simulink model "RadarSimulinkProjectRev009"  (R2024a)
settings: Solver=VariableStepAuto  StartTime=0.0  StopTime=0.0125  RelTol=1e-3
values from neighbouring files (symbols this model uses):
  AngleTime = SweepTime/10    (= 10000)    [InitializationOfVariables.m]    (also in InitializationOfVariablesRev000.m; InitializationOfVariablesRev001.m; InitializationOfVariablesRev003.m = 2097152; InitializationOfVariablesRev004.m = 2097152)
  ASR_LUT = Rsamp-OffsetDelayR    [InitializationOfVariablesRev003.m]    (also in InitializationOfVariablesRev004.m = round((R*2*SystemFs)/c))
  Btn_Debounce = 20000    [InitializationOfVariablesRev003.m]    (also in InitializationOfVariablesRev004.m)
  ChirpNc = 128    [InitializationOfVariablesRev003.m]    (also in InitializationOfVariablesRev004.m)
  ChirpSizeLength = FreqDeltaPeriod*361    (= 16245)    [InitializationOfVariablesRev003.m]    (also in InitializationOfVariablesRev004.m = 16384)
  DeciFactor = 8    [InitializationOfVariablesRev004.m]
  FCW = [FCW_p1, FCW_p2]    [InitializationOfVariablesRev003.m]    (also in InitializationOfVariablesRev004.m = f / SystemFs)
  RXFFTLength = 16384    [InitializationOfVariablesRev003.m]    (also in InitializationOfVariablesRev004.m = 2048)
  SweepTime = 100000    [InitializationOfVariables.m]    (also in InitializationOfVariablesRev000.m; InitializationOfVariablesRev001.m; InitializationOfVariablesRev003.m = 23068672; InitializationOfVariablesRev004.m = 23068672)
undefined symbols (not defined in the file or in its folder): SignalGenerationForAnalysis, Subsystem, xc7a200tfbg676
libraries: hdlBasic x407, hdlUtilities x11, hdlDSPIP x11, vmcUtilities x1
(part 4 of 4)

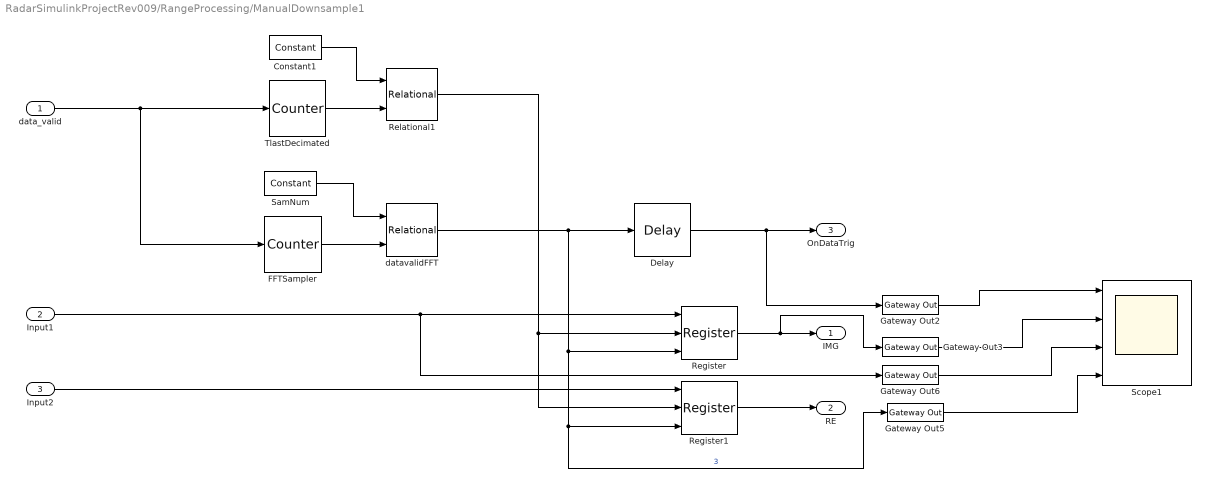
== system RadarSimulinkProjectRev009/RangeProcessing/ManualDownsample1 ==
  data_valid : Inport
  Input1 : Inport  Port=2
  Input2 : Inport  Port=3
  Constant1 : hdlBasic/Constant  const=RXFFTLength*8-1  gui_display_data_type=Fixed-point  arith_type=Signed (2's comp)  n_bits=16  bin_pt=0  preci_type=Single  exp_width=8  frac_width=24  explicit_period=off  period=1  XmcBlockStatus=1  maskContainerNames=tabcontainer1  block_type=constant  block_config=sysgen:Constant_config
  Delay : hdlBasic/Delay  rst=off  en=off  latency=1  reg_retiming=off  XmcBlockStatus=1  maskContainerNames=group1  block_type=delay  block_config=sysgen:Delay_config
  FFTSampler : hdlBasic/Counter  cnt_type=Count limited  cnt_to=DeciFactor-1  operation=Up  start_count=0  cnt_by_val=1  arith_type=Unsigned  n_bits=4  bin_pt=0  load_pin=off  rst=off  en=on  explicit_period=Explicit  period=P1  use_behavioral_HDL=off  implementation=Fabric  XmcBlockStatus=1  maskContainerNames=group1  block_type=counter  block_config=sysgen:Counter_config  block_width=531  block_height=1023
  Gateway Out{2..3,5..6} (4 alike) : hdlBasic/Gateway Out  inherit_from_input=off  bool_to_boolean=off  hdl_port=on  rows=1  columns=1  UseAsDAC=off  DACChannel='1'  interface=None  automatic_assignment=on  address_offset=hex2dec('00')  intf_name=''  intf_description=''  timing_constraint=None  locs_specified=off  LOCs={}  io_standard={}  XmcBlockStatus=1  maskContainerNames=group4  block_type=gatewayout  block_config=sysgen:gateway_out_config  block_width_w=590  block_height_w=620  block_width=620  block_height=750
  Register : hdlBasic/Register  init=0  rst=on  en=on  XmcBlockStatus=1  maskContainerNames=tabcontainer1  block_type=register  block_config=sysgen:Register_config
  Register1 : hdlBasic/Register  init=0  rst=on  en=on  XmcBlockStatus=1  maskContainerNames=tabcontainer1  block_type=register  block_config=sysgen:Register_config
  Relational1 : hdlBasic/Relational  mode=a=b  op_type=Bool  en=off  latency=0  XmcBlockStatus=1  maskContainerNames=tabcontainer1  block_type=relational  block_config=sysgen:Relational_config
  SamNum : hdlBasic/Constant  const=5  gui_display_data_type=Fixed-point  arith_type=Signed (2's comp)  n_bits=5  bin_pt=0  preci_type=Single  exp_width=8  frac_width=24  explicit_period=off  period=1  XmcBlockStatus=1  maskContainerNames=tabcontainer1  block_type=constant  block_config=sysgen:Constant_config
  Scope1 : Scope  NumInputPorts=4
  TlastDecimated : hdlBasic/Counter  cnt_type=Count limited  cnt_to=2047  operation=Up  start_count=0  cnt_by_val=1  arith_type=Unsigned  n_bits=12  bin_pt=0  load_pin=off  rst=off  en=on  explicit_period=Inferred from inputs  period=P1  use_behavioral_HDL=off  implementation=Fabric  XmcBlockStatus=1  maskContainerNames=group1  block_type=counter  block_config=sysgen:Counter_config  block_width=531  block_height=1023
  datavalidFFT : hdlBasic/Relational  mode=a=b  op_type=Bool  en=off  latency=0  XmcBlockStatus=1  maskContainerNames=tabcontainer1  block_type=relational  block_config=sysgen:Relational_config
  IMG : Outport
  RE : Outport  Port=2
  OnDataTrig : Outport  Port=3
  wires:
  data_valid/1 -> FFTSampler/1, TlastDecimated/1
  Constant1/1 -> Relational1/1
  FFTSampler/1 -> datavalidFFT/2
  datavalidFFT/1 -> Gateway Out5/1, Register1/3, Register/3, Delay/1  "3"
  TlastDecimated/1 -> Relational1/2
  SamNum/1 -> datavalidFFT/1
  Register/1 -> Gateway Out3/1, IMG/1
  Register1/1 -> RE/1
  Delay/1 -> Gateway Out2/1, OnDataTrig/1
  Input1/1 -> Gateway Out6/1, Register/1
  Input2/1 -> Register1/1
  Relational1/1 -> Register/2, Register1/2
  Gateway Out3/1 -> Scope1/2
  Gateway Out6/1 -> Scope1/3
  Gateway Out5/1 -> Scope1/4
  Gateway Out2/1 -> Scope1/1

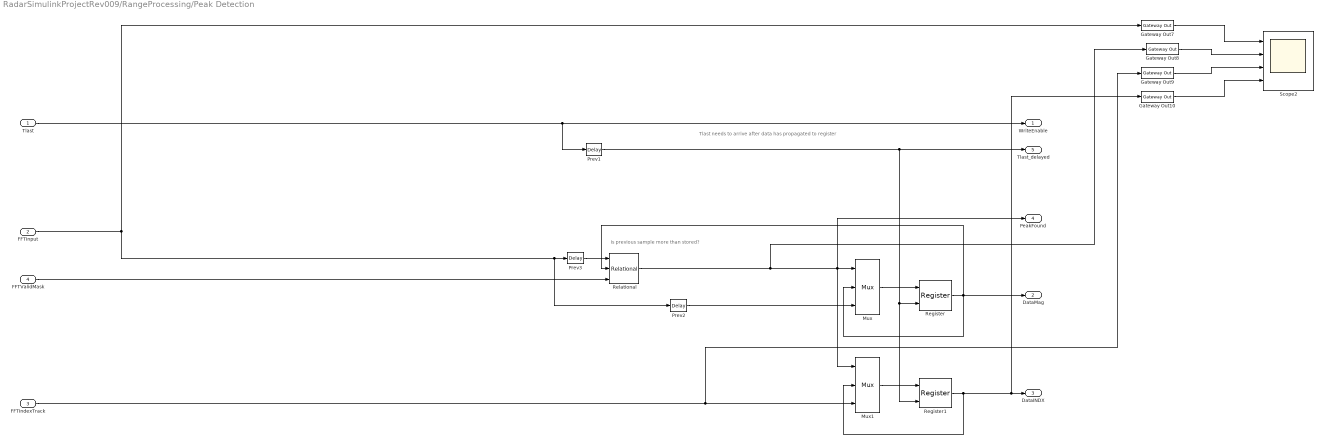
== system RadarSimulinkProjectRev009/RangeProcessing/Peak Detection ==
  note: Tlast needs to arrive after data has propagated to register
  note: Is previous sample more than stored?
  Tlast : Inport
  FFTInput : Inport  Port=2
  FFTIndexTrack : Inport  Port=3
  FFTValidMask : Inport  Port=4
  Gateway Out{7..10} (4 alike) : hdlBasic/Gateway Out  inherit_from_input=off  bool_to_boolean=off  hdl_port=on  rows=1  columns=1  UseAsDAC=off  DACChannel='1'  interface=None  automatic_assignment=on  address_offset=hex2dec('00')  intf_name=''  intf_description=''  timing_constraint=None  locs_specified=off  LOCs={}  io_standard={}  XmcBlockStatus=1  maskContainerNames=group4  block_type=gatewayout  block_config=sysgen:gateway_out_config  block_width_w=590  block_height_w=620  block_width=620  block_height=750
  Mux : hdlBasic/Mux  inputs=2  en=off  latency=0  precision=Full  arith_type=Unsigned  n_bits=16  bin_pt=14  quantization=Truncate  overflow=Wrap  XmcBlockStatus=1  maskContainerNames=tabcontainer1  block_type=mux  block_config=sysgen:Mux_config
  Mux1 : hdlBasic/Mux  inputs=2  en=off  latency=0  precision=Full  arith_type=Unsigned  n_bits=16  bin_pt=14  quantization=Truncate  overflow=Wrap  XmcBlockStatus=1  maskContainerNames=tabcontainer1  block_type=mux  block_config=sysgen:Mux_config
  Prev1 : hdlBasic/Delay  rst=off  en=off  latency=4  reg_retiming=off  XmcBlockStatus=1  maskContainerNames=group1  block_type=delay  block_config=sysgen:Delay_config
  Prev2 : hdlBasic/Delay  rst=off  en=off  latency=2  reg_retiming=off  XmcBlockStatus=1  maskContainerNames=group1  block_type=delay  block_config=sysgen:Delay_config
  Prev3 : hdlBasic/Delay  rst=off  en=off  latency=1  reg_retiming=off  XmcBlockStatus=1  maskContainerNames=group1  block_type=delay  block_config=sysgen:Delay_config
  Register : hdlBasic/Register  init=0  rst=on  en=off  XmcBlockStatus=1  maskContainerNames=tabcontainer1  block_type=register  block_config=sysgen:Register_config
  Register1 : hdlBasic/Register  init=0  rst=on  en=off  XmcBlockStatus=1  maskContainerNames=tabcontainer1  block_type=register  block_config=sysgen:Register_config
  Relational : hdlBasic/Relational  mode=a>b  op_type=Bool  en=on  latency=1  XmcBlockStatus=1  maskContainerNames=tabcontainer1  block_type=relational  block_config=sysgen:Relational_config
  Scope2 : Scope  NumInputPorts=4
  WriteEnable : Outport
  DataMag : Outport  Port=2
  DataINDX : Outport  Port=3
  PeakFound : Outport  Port=4
  Tlast_delayed : Outport  Port=5
  wires:
  FFTValidMask/1 -> Relational/3
  Tlast/1 -> Prev1/1, WriteEnable/1
  Prev2/1 -> Mux/3
  Register/1 -> Relational/2, DataMag/1, Mux/2
  Mux/1 -> Register/1
  Register1/1 -> Gateway Out10/1, DataINDX/1, Mux1/2
  FFTIndexTrack/1 -> Gateway Out9/1, Mux1/3
  Mux1/1 -> Register1/1
  Prev1/1 -> Register1/2, Register/2, Tlast_delayed/1
  Gateway Out7/1 -> Scope2/1
  Gateway Out8/1 -> Scope2/2
  Gateway Out9/1 -> Scope2/3
  Gateway Out10/1 -> Scope2/4
  FFTInput/1 -> Gateway Out7/1, Prev3/1, Prev2/1
  Prev3/1 -> Relational/1
  Relational/1 -> Gateway Out8/1, Mux1/1, Mux/1, PeakFound/1

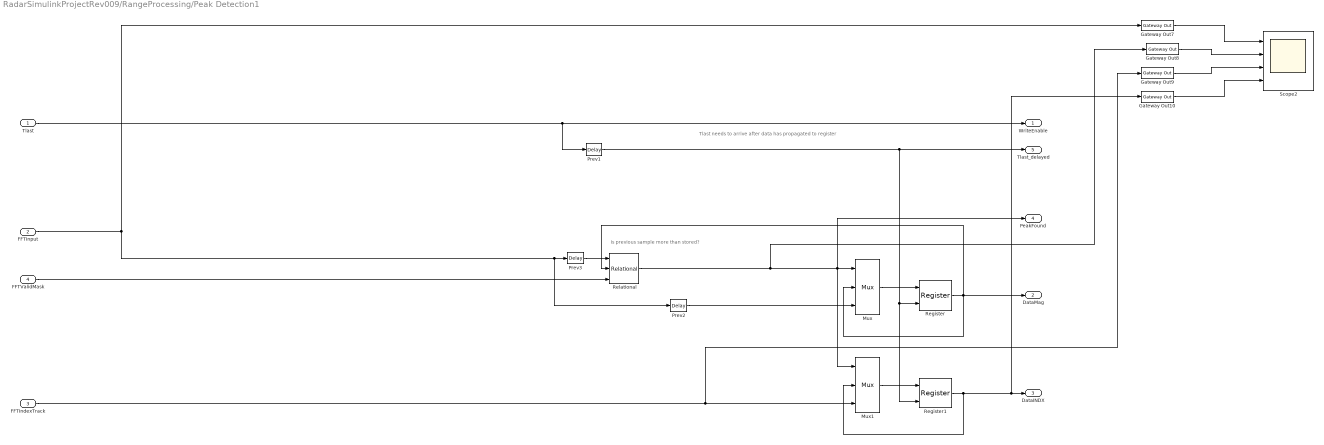
== system RadarSimulinkProjectRev009/RangeProcessing/Peak Detection1 ==
  note: Tlast needs to arrive after data has propagated to register
  note: Is previous sample more than stored?
  Tlast : Inport
  FFTInput : Inport  Port=2
  FFTIndexTrack : Inport  Port=3
  FFTValidMask : Inport  Port=4
  Gateway Out{7..10} (4 alike) : hdlBasic/Gateway Out  inherit_from_input=off  bool_to_boolean=off  hdl_port=on  rows=1  columns=1  UseAsDAC=off  DACChannel='1'  interface=None  automatic_assignment=on  address_offset=hex2dec('00')  intf_name=''  intf_description=''  timing_constraint=None  locs_specified=off  LOCs={}  io_standard={}  XmcBlockStatus=1  maskContainerNames=group4  block_type=gatewayout  block_config=sysgen:gateway_out_config  block_width_w=590  block_height_w=620  block_width=620  block_height=750
  Mux : hdlBasic/Mux  inputs=2  en=off  latency=0  precision=Full  arith_type=Unsigned  n_bits=16  bin_pt=14  quantization=Truncate  overflow=Wrap  XmcBlockStatus=1  maskContainerNames=tabcontainer1  block_type=mux  block_config=sysgen:Mux_config
  Mux1 : hdlBasic/Mux  inputs=2  en=off  latency=0  precision=Full  arith_type=Unsigned  n_bits=16  bin_pt=14  quantization=Truncate  overflow=Wrap  XmcBlockStatus=1  maskContainerNames=tabcontainer1  block_type=mux  block_config=sysgen:Mux_config
  Prev1 : hdlBasic/Delay  rst=off  en=off  latency=4  reg_retiming=off  XmcBlockStatus=1  maskContainerNames=group1  block_type=delay  block_config=sysgen:Delay_config
  Prev2 : hdlBasic/Delay  rst=off  en=off  latency=2  reg_retiming=off  XmcBlockStatus=1  maskContainerNames=group1  block_type=delay  block_config=sysgen:Delay_config
  Prev3 : hdlBasic/Delay  rst=off  en=off  latency=1  reg_retiming=off  XmcBlockStatus=1  maskContainerNames=group1  block_type=delay  block_config=sysgen:Delay_config
  Register : hdlBasic/Register  init=0  rst=on  en=off  XmcBlockStatus=1  maskContainerNames=tabcontainer1  block_type=register  block_config=sysgen:Register_config
  Register1 : hdlBasic/Register  init=0  rst=on  en=off  XmcBlockStatus=1  maskContainerNames=tabcontainer1  block_type=register  block_config=sysgen:Register_config
  Relational : hdlBasic/Relational  mode=a>b  op_type=Bool  en=on  latency=1  XmcBlockStatus=1  maskContainerNames=tabcontainer1  block_type=relational  block_config=sysgen:Relational_config
  Scope2 : Scope  NumInputPorts=4
  WriteEnable : Outport
  DataMag : Outport  Port=2
  DataINDX : Outport  Port=3
  PeakFound : Outport  Port=4
  Tlast_delayed : Outport  Port=5
  wires:
  FFTValidMask/1 -> Relational/3
  Tlast/1 -> Prev1/1, WriteEnable/1
  Prev2/1 -> Mux/3
  Register/1 -> Relational/2, DataMag/1, Mux/2
  Mux/1 -> Register/1
  Register1/1 -> Gateway Out10/1, DataINDX/1, Mux1/2
  FFTIndexTrack/1 -> Gateway Out9/1, Mux1/3
  Mux1/1 -> Register1/1
  Prev1/1 -> Register1/2, Register/2, Tlast_delayed/1
  Gateway Out7/1 -> Scope2/1
  Gateway Out8/1 -> Scope2/2
  Gateway Out9/1 -> Scope2/3
  Gateway Out10/1 -> Scope2/4
  FFTInput/1 -> Gateway Out7/1, Prev3/1, Prev2/1
  Prev3/1 -> Relational/1
  Relational/1 -> Gateway Out8/1, Mux1/1, Mux/1, PeakFound/1

== system RadarSimulinkProjectRev009/RangeProcessing/RX Lowpass Filter ==
  validIN : Inport
  dataIN : Inport  Port=2
  Convert10 : hdlBasic/Convert  gui_display_data_type=Fixed-point  arith_type=Signed (2's comp)  n_bits=32  bin_pt=16  float_type=Single  exp_bits=8  fraction_bits=24  quantization="Round  (unbiased: Even Values)"  overflow=Saturate  en=off  latency=1  pipeline=off  XmcBlockStatus=1  maskContainerNames=group2  block_type=convert  block_config=sysgen:Convert_config  block_width=595  block_height=885
  Convert12 : hdlBasic/Convert  gui_display_data_type=Fixed-point  arith_type=Signed (2's comp)  n_bits=32  bin_pt=16  float_type=Single  exp_bits=8  fraction_bits=24  quantization="Round  (unbiased: Even Values)"  overflow=Saturate  en=off  latency=1  pipeline=off  XmcBlockStatus=1  maskContainerNames=group2  block_type=convert  block_config=sysgen:Convert_config  block_width=595  block_height=885
  Delay : hdlBasic/Delay  rst=off  en=off  latency=450  reg_retiming=off  XmcBlockStatus=1  maskContainerNames=group1  block_type=delay  block_config=sysgen:Delay_config
  Digital FIR Filter6 : hdlBasic/Digital FIR Filter  coeff_source=off  coefficientvector=b1  coeff_calulate=on  coefficient_width=13  coefficient_fractional_bits=13  interpolation_filter_rate=1  decimation_filter_rate=4  fda_coefficientvector=[-0.0024 -0.0042 0.0095 0.0200 -0.0380 -0.0696 0.1374 0.4472 0.4472 0.1374 -0.0696 -0.0380 0.0200 0.0095 -0.0042 -0.0024]  simulation_type=fast_sim  simulation_model=sysgen:fir_macro  XmcBlockStatus=1  maskContainerNames=group1  block_type=fir_macro  block_config=sysgen:fir_macro_config
  Digital FIR Filter7 : hdlBasic/Digital FIR Filter  coeff_source=off  coefficientvector=b2  coeff_calulate=on  coefficient_width=13  coefficient_fractional_bits=13  interpolation_filter_rate=1  decimation_filter_rate=4  fda_coefficientvector=[-0.0024 -0.0042 0.0095 0.0200 -0.0380 -0.0696 0.1374 0.4472 0.4472 0.1374 -0.0696 -0.0380 0.0200 0.0095 -0.0042 -0.0024]  simulation_type=fast_sim  simulation_model=sysgen:fir_macro  XmcBlockStatus=1  maskContainerNames=group1  block_type=fir_macro  block_config=sysgen:fir_macro_config
  Digital FIR Filter8 : hdlBasic/Digital FIR Filter  coeff_source=off  coefficientvector=b3  coeff_calulate=on  coefficient_width=2  coefficient_fractional_bits=2  interpolation_filter_rate=1  decimation_filter_rate=1  fda_coefficientvector=[-0.0024 -0.0042 0.0095 0.0200 -0.0380 -0.0696 0.1374 0.4472 0.4472 0.1374 -0.0696 -0.0380 0.0200 0.0095 -0.0042 -0.0024]  simulation_type=fast_sim  simulation_model=sysgen:fir_macro  XmcBlockStatus=1  maskContainerNames=group1  block_type=fir_macro  block_config=sysgen:fir_macro_config
  tready : Outport
  dataOUT : Outport  Port=2
  wires:
  Convert12/1 -> Digital FIR Filter8/1
  Digital FIR Filter6/1 -> Convert10/1
  Digital FIR Filter7/1 -> Convert12/1
  Convert10/1 -> Digital FIR Filter7/1
  Digital FIR Filter8/1 -> dataOUT/1
  dataIN/1 -> Digital FIR Filter6/1
  validIN/1 -> Delay/1
  Delay/1 -> tready/1

== system RadarSimulinkProjectRev009/RangeProcessing/RX Lowpass Filter1 ==
  dataIN : Inport
  Convert10 : hdlBasic/Convert  gui_display_data_type=Fixed-point  arith_type=Signed (2's comp)  n_bits=32  bin_pt=16  float_type=Single  exp_bits=8  fraction_bits=24  quantization="Round  (unbiased: Even Values)"  overflow=Saturate  en=off  latency=1  pipeline=off  XmcBlockStatus=1  maskContainerNames=group2  block_type=convert  block_config=sysgen:Convert_config  block_width=595  block_height=885
  Convert12 : hdlBasic/Convert  gui_display_data_type=Fixed-point  arith_type=Signed (2's comp)  n_bits=32  bin_pt=16  float_type=Single  exp_bits=8  fraction_bits=24  quantization="Round  (unbiased: Even Values)"  overflow=Saturate  en=off  latency=1  pipeline=off  XmcBlockStatus=1  maskContainerNames=group2  block_type=convert  block_config=sysgen:Convert_config  block_width=595  block_height=885
  Digital FIR Filter6 : hdlBasic/Digital FIR Filter  coeff_source=off  coefficientvector=b1  coeff_calulate=on  coefficient_width=13  coefficient_fractional_bits=13  interpolation_filter_rate=1  decimation_filter_rate=4  fda_coefficientvector=[-0.0024 -0.0042 0.0095 0.0200 -0.0380 -0.0696 0.1374 0.4472 0.4472 0.1374 -0.0696 -0.0380 0.0200 0.0095 -0.0042 -0.0024]  simulation_type=fast_sim  simulation_model=sysgen:fir_macro  XmcBlockStatus=1  maskContainerNames=group1  block_type=fir_macro  block_config=sysgen:fir_macro_config
  Digital FIR Filter7 : hdlBasic/Digital FIR Filter  coeff_source=off  coefficientvector=b2  coeff_calulate=on  coefficient_width=13  coefficient_fractional_bits=13  interpolation_filter_rate=1  decimation_filter_rate=4  fda_coefficientvector=[-0.0024 -0.0042 0.0095 0.0200 -0.0380 -0.0696 0.1374 0.4472 0.4472 0.1374 -0.0696 -0.0380 0.0200 0.0095 -0.0042 -0.0024]  simulation_type=fast_sim  simulation_model=sysgen:fir_macro  XmcBlockStatus=1  maskContainerNames=group1  block_type=fir_macro  block_config=sysgen:fir_macro_config
  Digital FIR Filter8 : hdlBasic/Digital FIR Filter  coeff_source=off  coefficientvector=b3  coeff_calulate=on  coefficient_width=13  coefficient_fractional_bits=13  interpolation_filter_rate=1  decimation_filter_rate=1  fda_coefficientvector=[-0.0024 -0.0042 0.0095 0.0200 -0.0380 -0.0696 0.1374 0.4472 0.4472 0.1374 -0.0696 -0.0380 0.0200 0.0095 -0.0042 -0.0024]  simulation_type=fast_sim  simulation_model=sysgen:fir_macro  XmcBlockStatus=1  maskContainerNames=group1  block_type=fir_macro  block_config=sysgen:fir_macro_config
  dataOUT : Outport
  wires:
  Convert12/1 -> Digital FIR Filter8/1
  Digital FIR Filter6/1 -> Convert10/1
  Digital FIR Filter7/1 -> Convert12/1
  Convert10/1 -> Digital FIR Filter7/1
  Digital FIR Filter8/1 -> dataOUT/1
  dataIN/1 -> Digital FIR Filter6/1

== system RadarSimulinkProjectRev009/RangeProcessing/RX Lowpass Filter2 ==
  dataIN : Inport
  Convert10 : hdlBasic/Convert  gui_display_data_type=Fixed-point  arith_type=Signed (2's comp)  n_bits=32  bin_pt=16  float_type=Single  exp_bits=8  fraction_bits=24  quantization="Round  (unbiased: Even Values)"  overflow=Saturate  en=off  latency=1  pipeline=off  XmcBlockStatus=1  maskContainerNames=group2  block_type=convert  block_config=sysgen:Convert_config  block_width=595  block_height=885
  Convert12 : hdlBasic/Convert  gui_display_data_type=Fixed-point  arith_type=Signed (2's comp)  n_bits=32  bin_pt=16  float_type=Single  exp_bits=8  fraction_bits=24  quantization="Round  (unbiased: Even Values)"  overflow=Saturate  en=off  latency=1  pipeline=off  XmcBlockStatus=1  maskContainerNames=group2  block_type=convert  block_config=sysgen:Convert_config  block_width=595  block_height=885
  Digital FIR Filter6 : hdlBasic/Digital FIR Filter  coeff_source=off  coefficientvector=b1  coeff_calulate=on  coefficient_width=13  coefficient_fractional_bits=13  interpolation_filter_rate=1  decimation_filter_rate=4  fda_coefficientvector=[-0.0024 -0.0042 0.0095 0.0200 -0.0380 -0.0696 0.1374 0.4472 0.4472 0.1374 -0.0696 -0.0380 0.0200 0.0095 -0.0042 -0.0024]  simulation_type=fast_sim  simulation_model=sysgen:fir_macro  XmcBlockStatus=1  maskContainerNames=group1  block_type=fir_macro  block_config=sysgen:fir_macro_config
  Digital FIR Filter7 : hdlBasic/Digital FIR Filter  coeff_source=off  coefficientvector=b2  coeff_calulate=on  coefficient_width=13  coefficient_fractional_bits=13  interpolation_filter_rate=1  decimation_filter_rate=4  fda_coefficientvector=[-0.0024 -0.0042 0.0095 0.0200 -0.0380 -0.0696 0.1374 0.4472 0.4472 0.1374 -0.0696 -0.0380 0.0200 0.0095 -0.0042 -0.0024]  simulation_type=fast_sim  simulation_model=sysgen:fir_macro  XmcBlockStatus=1  maskContainerNames=group1  block_type=fir_macro  block_config=sysgen:fir_macro_config
  Digital FIR Filter8 : hdlBasic/Digital FIR Filter  coeff_source=off  coefficientvector=b3  coeff_calulate=on  coefficient_width=2  coefficient_fractional_bits=2  interpolation_filter_rate=1  decimation_filter_rate=1  fda_coefficientvector=[-0.0024 -0.0042 0.0095 0.0200 -0.0380 -0.0696 0.1374 0.4472 0.4472 0.1374 -0.0696 -0.0380 0.0200 0.0095 -0.0042 -0.0024]  simulation_type=fast_sim  simulation_model=sysgen:fir_macro  XmcBlockStatus=1  maskContainerNames=group1  block_type=fir_macro  block_config=sysgen:fir_macro_config
  dataOUT : Outport
  wires:
  Convert12/1 -> Digital FIR Filter8/1
  Digital FIR Filter6/1 -> Convert10/1
  Digital FIR Filter7/1 -> Convert12/1
  Convert10/1 -> Digital FIR Filter7/1
  Digital FIR Filter8/1 -> dataOUT/1
  dataIN/1 -> Digital FIR Filter6/1

== system RadarSimulinkProjectRev009/RangeProcessing/RX Lowpass Filter3 ==
  dataIN : Inport
  Convert10 : hdlBasic/Convert  gui_display_data_type=Fixed-point  arith_type=Signed (2's comp)  n_bits=32  bin_pt=16  float_type=Single  exp_bits=8  fraction_bits=24  quantization="Round  (unbiased: Even Values)"  overflow=Saturate  en=off  latency=1  pipeline=off  XmcBlockStatus=1  maskContainerNames=group2  block_type=convert  block_config=sysgen:Convert_config  block_width=595  block_height=885
  Convert12 : hdlBasic/Convert  gui_display_data_type=Fixed-point  arith_type=Signed (2's comp)  n_bits=32  bin_pt=16  float_type=Single  exp_bits=8  fraction_bits=24  quantization="Round  (unbiased: Even Values)"  overflow=Saturate  en=off  latency=1  pipeline=off  XmcBlockStatus=1  maskContainerNames=group2  block_type=convert  block_config=sysgen:Convert_config  block_width=595  block_height=885
  Digital FIR Filter6 : hdlBasic/Digital FIR Filter  coeff_source=off  coefficientvector=b1  coeff_calulate=on  coefficient_width=13  coefficient_fractional_bits=13  interpolation_filter_rate=1  decimation_filter_rate=4  fda_coefficientvector=[-0.0024 -0.0042 0.0095 0.0200 -0.0380 -0.0696 0.1374 0.4472 0.4472 0.1374 -0.0696 -0.0380 0.0200 0.0095 -0.0042 -0.0024]  simulation_type=fast_sim  simulation_model=sysgen:fir_macro  XmcBlockStatus=1  maskContainerNames=group1  block_type=fir_macro  block_config=sysgen:fir_macro_config
  Digital FIR Filter7 : hdlBasic/Digital FIR Filter  coeff_source=off  coefficientvector=b2  coeff_calulate=on  coefficient_width=13  coefficient_fractional_bits=13  interpolation_filter_rate=1  decimation_filter_rate=4  fda_coefficientvector=[-0.0024 -0.0042 0.0095 0.0200 -0.0380 -0.0696 0.1374 0.4472 0.4472 0.1374 -0.0696 -0.0380 0.0200 0.0095 -0.0042 -0.0024]  simulation_type=fast_sim  simulation_model=sysgen:fir_macro  XmcBlockStatus=1  maskContainerNames=group1  block_type=fir_macro  block_config=sysgen:fir_macro_config
  Digital FIR Filter8 : hdlBasic/Digital FIR Filter  coeff_source=off  coefficientvector=b3  coeff_calulate=on  coefficient_width=13  coefficient_fractional_bits=13  interpolation_filter_rate=1  decimation_filter_rate=1  fda_coefficientvector=[-0.0024 -0.0042 0.0095 0.0200 -0.0380 -0.0696 0.1374 0.4472 0.4472 0.1374 -0.0696 -0.0380 0.0200 0.0095 -0.0042 -0.0024]  simulation_type=fast_sim  simulation_model=sysgen:fir_macro  XmcBlockStatus=1  maskContainerNames=group1  block_type=fir_macro  block_config=sysgen:fir_macro_config
  dataOUT : Outport
  wires:
  Convert12/1 -> Digital FIR Filter8/1
  Digital FIR Filter6/1 -> Convert10/1
  Digital FIR Filter7/1 -> Convert12/1
  Convert10/1 -> Digital FIR Filter7/1
  Digital FIR Filter8/1 -> dataOUT/1
  dataIN/1 -> Digital FIR Filter6/1

== system RadarSimulinkProjectRev009/RangeProcessing/Subsystem ==
  note: For radix burst, tlast should come from each chirp end,
      | in this case, tlast triggers every 128 samples, (0, 2048, 4096..ect until 262,000th data point, then moves on to the next set at 1, 2049, 4097, ect.)
  note: Chirp*FFT=total data
      | 128*2048=262,000
  note: Needs to be 0, 1024, 2048
      | Then 1, 1025, 2049, ect
  tvalid : Inport
  Reset : Inport  Port=2
  Chirp : hdlBasic/Counter  cnt_type=Count limited  cnt_to=ChirpNc-1  operation=Up  start_count=0  cnt_by_val=1  arith_type=Unsigned  n_bits=8  bin_pt=0  load_pin=off  rst=on  en=on  explicit_period=Explicit  period=P1  use_behavioral_HDL=off  implementation=Fabric  XmcBlockStatus=1  maskContainerNames=group1  block_type=counter  block_config=sysgen:Counter_config  block_width=531  block_height=1023
  Constant : hdlBasic/Constant  const=ChirpNc-1  gui_display_data_type=Fixed-point  arith_type=Signed (2's comp)  n_bits=16  bin_pt=0  preci_type=Single  exp_width=8  frac_width=24  explicit_period=off  period=1  XmcBlockStatus=1  maskContainerNames=tabcontainer1  block_type=constant  block_config=sysgen:Constant_config
  Constant1 : hdlBasic/Constant  const=RXFFTLength  gui_display_data_type=Fixed-point  arith_type=Signed (2's comp)  n_bits=16  bin_pt=0  preci_type=Single  exp_width=8  frac_width=24  explicit_period=off  period=1  XmcBlockStatus=1  maskContainerNames=tabcontainer1  block_type=constant  block_config=sysgen:Constant_config
  FFT : hdlBasic/Counter  cnt_type=Count limited  cnt_to=RXFFTLength-1  operation=Up  start_count=0  cnt_by_val=1  arith_type=Unsigned  n_bits=13  bin_pt=0  load_pin=off  rst=on  en=on  explicit_period=Explicit  period=P1  use_behavioral_HDL=off  implementation=Fabric  XmcBlockStatus=1  maskContainerNames=group1  block_type=counter  block_config=sysgen:Counter_config  block_width=531  block_height=1023
  MultAdd : hdlBasic/MultAdd  mode=Addition  en=off  latency=0  precision=User Defined  arith_type=Unsigned  n_bits=18  bin_pt=0  XmcBlockStatus=1  maskContainerNames=tabcontainer1  block_type=multadd  block_config=sysgen:MultAdd_config
  Relational : hdlBasic/Relational  mode=a=b  op_type=Bool  en=off  latency=0  XmcBlockStatus=1  maskContainerNames=tabcontainer1  block_type=relational  block_config=sysgen:Relational_config
  AddrOut : Outport
  FFTtlast : Outport  Port=2
  wires:
  Reset/1 -> FFT/1, Chirp/1
  tvalid/1 -> Chirp/2
  Chirp/1 -> MultAdd/1, Relational/1
  Constant/1 -> Relational/2
  Relational/1 -> FFTtlast/1, FFT/2
  Constant1/1 -> MultAdd/2
  FFT/1 -> MultAdd/3
  MultAdd/1 -> AddrOut/1

== system RadarSimulinkProjectRev009/RangeProcessing/Subsystem1 ==
  RE : Inport
  IMG : Inport  Port=2
  Enable : EnablePort
  To Workspace : ToWorkspace  VariableName=REValues1  SampleTime=-1
  To Workspace1 : ToWorkspace  VariableName=IMGValues1  SampleTime=-1
  wires:
  IMG/1 -> To Workspace1/1
  RE/1 -> To Workspace/1

== system RadarSimulinkProjectRev009/Velocity Processing/FFTTracking ==
  note: Should restart counter at beggining or end,
      | In Radix mode, Tlast is not the beggining because there is a gap
  note: In Radix burst, this is active for only real frame of data
      | In Pipeline, it's always active
  note: Bring back to 0 at start
  data_Active : Inport
  StatusReady : Inport  Port=2
  IndexTracker : hdlBasic/Counter  cnt_type=Count limited  cnt_to=ChirpNc-1  operation=Up  start_count=0  cnt_by_val=1  arith_type=Unsigned  n_bits=14  bin_pt=0  load_pin=off  rst=on  en=on  explicit_period=Explicit  period=P1  use_behavioral_HDL=off  implementation=Fabric  XmcBlockStatus=1  maskContainerNames=group1  block_type=counter  block_config=sysgen:Counter_config  block_width=531  block_height=1023
  Inverter : hdlBasic/Inverter  en=off  latency=0  XmcBlockStatus=1  maskContainerNames=group2  block_type=inv  block_config=sysgen:Inverter_config
  Logical1 : hdlBasic/Logical  logical_function=AND  inputs=2  en=off  latency=0  precision=Full  arith_type=Unsigned  n_bits=16  bin_pt=0  align_bp=on  overflow=[]  quantization=[]  XmcBlockStatus=1  maskContainerNames=tabcontainer1  block_type=logical  block_config=sysgen:Logical_config
  FFTIndex : Outport
  PeakSerachEnable : Outport  Port=2
  wires:
  IndexTracker/1 -> FFTIndex/1
  Inverter/1 -> IndexTracker/1
  Logical1/1 -> PeakSerachEnable/1, IndexTracker/2
  StatusReady/1 -> Logical1/1, Inverter/1
  data_Active/1 -> Logical1/2

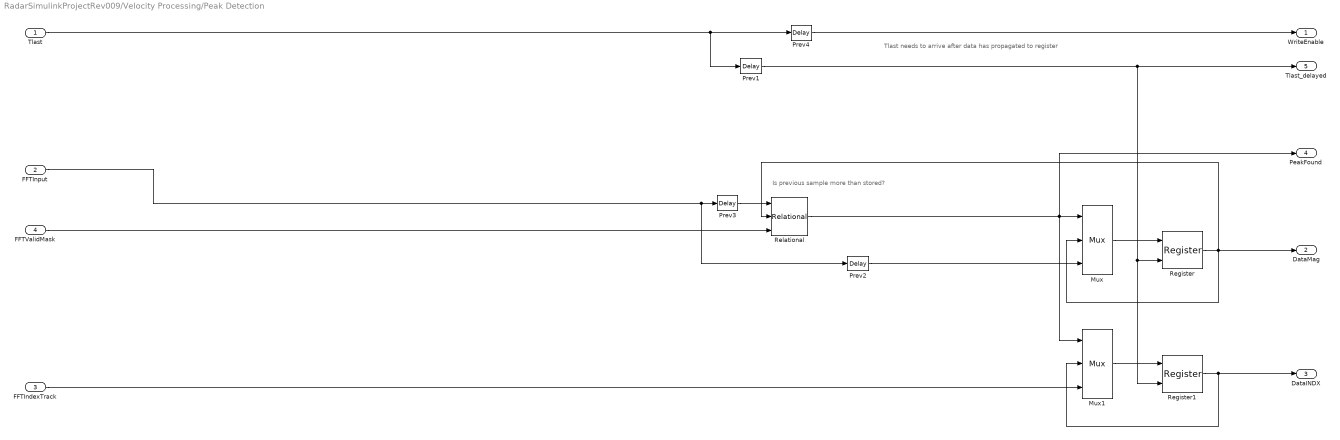
== system RadarSimulinkProjectRev009/Velocity Processing/Peak Detection ==
  note: Tlast needs to arrive after data has propagated to register
  note: Is previous sample more than stored?
  Tlast : Inport
  FFTInput : Inport  Port=2
  FFTIndexTrack : Inport  Port=3
  FFTValidMask : Inport  Port=4
  Mux : hdlBasic/Mux  inputs=2  en=off  latency=0  precision=Full  arith_type=Unsigned  n_bits=16  bin_pt=14  quantization=Truncate  overflow=Wrap  XmcBlockStatus=1  maskContainerNames=tabcontainer1  block_type=mux  block_config=sysgen:Mux_config
  Mux1 : hdlBasic/Mux  inputs=2  en=off  latency=0  precision=Full  arith_type=Unsigned  n_bits=16  bin_pt=14  quantization=Truncate  overflow=Wrap  XmcBlockStatus=1  maskContainerNames=tabcontainer1  block_type=mux  block_config=sysgen:Mux_config
  Prev1 : hdlBasic/Delay  rst=off  en=off  latency=3  reg_retiming=off  XmcBlockStatus=1  maskContainerNames=group1  block_type=delay  block_config=sysgen:Delay_config
  Prev2 : hdlBasic/Delay  rst=off  en=off  latency=2  reg_retiming=off  XmcBlockStatus=1  maskContainerNames=group1  block_type=delay  block_config=sysgen:Delay_config
  Prev3 : hdlBasic/Delay  rst=off  en=off  latency=1  reg_retiming=off  XmcBlockStatus=1  maskContainerNames=group1  block_type=delay  block_config=sysgen:Delay_config
  Prev4 : hdlBasic/Delay  rst=off  en=off  latency=3  reg_retiming=off  XmcBlockStatus=1  maskContainerNames=group1  block_type=delay  block_config=sysgen:Delay_config
  Register : hdlBasic/Register  init=0  rst=on  en=off  XmcBlockStatus=1  maskContainerNames=tabcontainer1  block_type=register  block_config=sysgen:Register_config
  Register1 : hdlBasic/Register  init=0  rst=on  en=off  XmcBlockStatus=1  maskContainerNames=tabcontainer1  block_type=register  block_config=sysgen:Register_config
  Relational : hdlBasic/Relational  mode=a>b  op_type=Bool  en=on  latency=1  XmcBlockStatus=1  maskContainerNames=tabcontainer1  block_type=relational  block_config=sysgen:Relational_config
  WriteEnable : Outport
  DataMag : Outport  Port=2
  DataINDX : Outport  Port=3
  PeakFound : Outport  Port=4
  Tlast_delayed : Outport  Port=5
  wires:
  FFTValidMask/1 -> Relational/3
  Tlast/1 -> Prev1/1, Prev4/1
  Prev2/1 -> Mux/3
  Register/1 -> Relational/2, DataMag/1, Mux/2
  Mux/1 -> Register/1
  Register1/1 -> DataINDX/1, Mux1/2
  FFTIndexTrack/1 -> Mux1/3
  Mux1/1 -> Register1/1
  Prev1/1 -> Register1/2, Register/2, Tlast_delayed/1
  FFTInput/1 -> Prev3/1, Prev2/1
  Prev3/1 -> Relational/1
  Relational/1 -> Mux1/1, Mux/1, PeakFound/1
  Prev4/1 -> WriteEnable/1

== system RadarSimulinkProjectRev009/Velocity Processing/Peak Detection1 ==
  note: Tlast needs to arrive after data has propagated to register
  note: Is previous sample more than stored?
  Tlast : Inport
  FFTInput : Inport  Port=2
  FFTIndexTrack : Inport  Port=3
  FFTValidMask : Inport  Port=4
  Mux : hdlBasic/Mux  inputs=2  en=off  latency=0  precision=Full  arith_type=Unsigned  n_bits=16  bin_pt=14  quantization=Truncate  overflow=Wrap  XmcBlockStatus=1  maskContainerNames=tabcontainer1  block_type=mux  block_config=sysgen:Mux_config
  Mux1 : hdlBasic/Mux  inputs=2  en=off  latency=0  precision=Full  arith_type=Unsigned  n_bits=16  bin_pt=14  quantization=Truncate  overflow=Wrap  XmcBlockStatus=1  maskContainerNames=tabcontainer1  block_type=mux  block_config=sysgen:Mux_config
  Prev1 : hdlBasic/Delay  rst=off  en=off  latency=4  reg_retiming=off  XmcBlockStatus=1  maskContainerNames=group1  block_type=delay  block_config=sysgen:Delay_config
  Prev2 : hdlBasic/Delay  rst=off  en=off  latency=2  reg_retiming=off  XmcBlockStatus=1  maskContainerNames=group1  block_type=delay  block_config=sysgen:Delay_config
  Prev3 : hdlBasic/Delay  rst=off  en=off  latency=1  reg_retiming=off  XmcBlockStatus=1  maskContainerNames=group1  block_type=delay  block_config=sysgen:Delay_config
  Register : hdlBasic/Register  init=0  rst=on  en=off  XmcBlockStatus=1  maskContainerNames=tabcontainer1  block_type=register  block_config=sysgen:Register_config
  Register1 : hdlBasic/Register  init=0  rst=on  en=off  XmcBlockStatus=1  maskContainerNames=tabcontainer1  block_type=register  block_config=sysgen:Register_config
  Relational : hdlBasic/Relational  mode=a>b  op_type=Bool  en=on  latency=1  XmcBlockStatus=1  maskContainerNames=tabcontainer1  block_type=relational  block_config=sysgen:Relational_config
  WriteEnable : Outport
  DataMag : Outport  Port=2
  DataINDX : Outport  Port=3
  PeakFound : Outport  Port=4
  Tlast_delayed : Outport  Port=5
  wires:
  FFTValidMask/1 -> Relational/3
  Tlast/1 -> Prev1/1, WriteEnable/1
  Prev2/1 -> Mux/3
  Register/1 -> Relational/2, DataMag/1, Mux/2
  Mux/1 -> Register/1
  Register1/1 -> DataINDX/1, Mux1/2
  FFTIndexTrack/1 -> Mux1/3
  Mux1/1 -> Register1/1
  Prev1/1 -> Register1/2, Register/2, Tlast_delayed/1
  FFTInput/1 -> Prev3/1, Prev2/1
  Prev3/1 -> Relational/1
  Relational/1 -> Mux1/1, Mux/1, PeakFound/1

== matlab function RadarSimulinkProjectRev009/MATLAB Function ==
  data: a input; b input; c input; d input; ao output; noisePower input; bo output; co output; do output
function [ao,bo,co,do] = fcn(a,b,c,d,noisePower)
    noise = noisePower*randn(size(a));
    ao = real(a)+noise;
    bo = real(b)+noise;
    co = real(c)+noise;
    do = real(d)+noise;
end
